simulink model "mavsim_trim"  (R2017b)
settings: Solver=ode45  StartTime=0.0  StopTime=10000  RelTol=1e-3  EnableMultiTasking=on
undefined symbols (not defined in the file or in its folder): forces_moments, P
settings Model: Creator=beard  LastModifiedBy=jpaine
settings DataIOCC: LimitDataPoints=on  SaveFormat=Array  SignalLoggingSaveFormat=ModelDataLogs
settings OptimizationCC: ExpressionDepthLimit=2147483647  InitFltsAndDblsToZero=on  LifeSpan=inf
settings DebuggingCC: UnderspecifiedInitializationDetection=Classic  MergeDetectMultiDrivingBlocksExec=none  SolverPrmCheckMsg=warning  FcnCallInpInsideContextMsg=warning  StateNameClashWarn=warning  SFUnexpectedBacktrackingDiag=warning  SFNoUnconditionalDefaultTransitionDiag=warning  SFExecutionAtInitializationDiag=none
settings HardwareCC: ProdBitPerPointer=32  ProdBitPerSizeT=32  ProdBitPerPtrDiffT=32  ProdLargestAtomicFloat=None  ProdIntDivRoundTo=Undefined  ProdEndianess=Unspecified  ProdWordSize=32  ProdHWDeviceType=32-bit Generic
settings ModelReferenceCC: PropagateSignalLabelsOutOfModel=off
settings CodeAppCC: StateflowObjectComments=on
settings GRTTargetCC: TargetLangStandard=C89/C90 (ANSI)  GeneratePreprocessorConditionals=Disable all  CombineOutputUpdateFcns=off  GRTInterface=on
settings ConfigComp: CovMetricSettings=dw  CovHtmlReporting=on  CovSaveCumulativeToWorkspaceVar=on  CovSaveSingleToWorkspaceVar=on  CovExternalEMLEnable=off  CovSFcnEnable=off

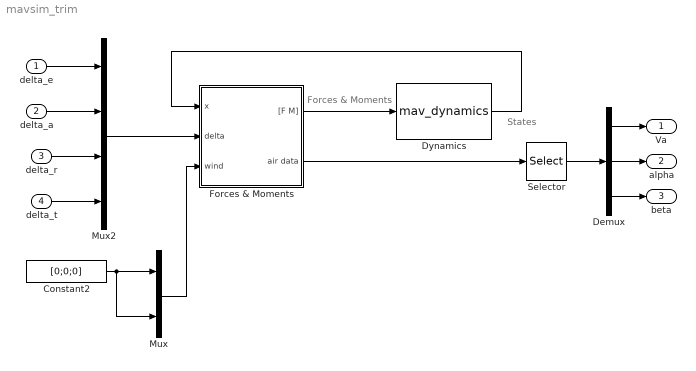
== system mavsim_trim ==
  note: Forces & Moments
  note: States
  delta_e : Inport
  delta_a : Inport  Port=2
  delta_r : Inport  Port=3
  delta_t : Inport  Port=4
  Constant2 : Constant  Value=[0;0;0]
  Demux : Demux  Outputs=3
  Dynamics : S-Function  FunctionName=mav_dynamics  Parameters=P  SFunctionDeploymentMode=off  EnableBusSupport=off
  Forces & Moments : Subsystem
  Mux : Mux  Inputs=2
  Mux2 : Mux
  Selector : Selector  InputPortWidth=6  IndexOptions=Index vector (dialog)  Indices=[1 2 3]  OutputSizes=1
  Va : Outport
  alpha : Outport  Port=2
  beta : Outport  Port=3
  wires:
  Constant2/1 -> Mux/1, Mux/2
  delta_e/1 -> Mux2/1
  delta_a/1 -> Mux2/2
  delta_r/1 -> Mux2/3
  delta_t/1 -> Mux2/4
  Dynamics/1 -> Forces & Moments/1(x)
  Mux2/1 -> Forces & Moments/2(delta)
  Forces & Moments/1("[F M]") -> Dynamics/1
  Mux/1 -> Forces & Moments/3(wind)
  Forces & Moments/2(air data) -> Selector/1
  Selector/1 -> Demux/1
  Demux/1 -> Va/1
  Demux/2 -> alpha/1
  Demux/3 -> beta/1

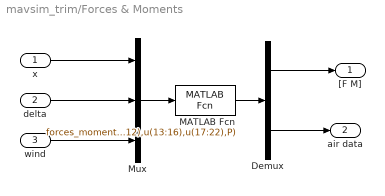
== system mavsim_trim/Forces & Moments ==
  x : Inport
  delta : Inport  Port=2
  wind : Inport  Port=3
  Demux : Demux  Outputs=[6;6]
  MATLAB Fcn : MATLABFcn  MATLABFcn=forces_moments(u(1:12),u(13:16),u(17:22),P)  OutputDimensions=12
  Mux : Mux  Inputs=3
  "[F M]" : Outport
  air data : Outport  Port=2
  wires:
  Demux/2 -> air data/1
  Mux/1 -> MATLAB Fcn/1
  Demux/1 -> "[F M]"/1
  MATLAB Fcn/1 -> Demux/1
  wind/1 -> Mux/3
  delta/1 -> Mux/2
  x/1 -> Mux/1
